simulink model "gm_sine_wave"  (R2020a)
settings: Solver=VariableStepAuto  StartTime=0.0  StopTime=1e-3  RelTol=1e-3
undefined symbols (not defined in the file or in its folder): amplitud, main_frequency, PLL_FREQUENCY
libraries: dspsrcs4 x1
settings Model: Creator=giova  LastModifiedBy=giova
settings OptimizationCC: BlockReduction=off  ConditionallyExecuteInputs=off
settings DebuggingCC: InheritedTsInSrcMsg=none

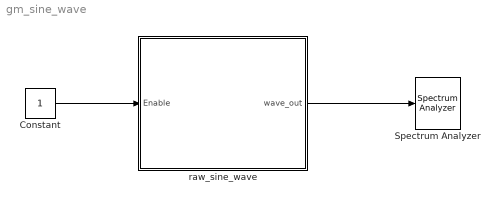
== system gm_sine_wave ==
  Constant : Constant  OutDataTypeStr=boolean  SampleTime=-1
  Spectrum Analyzer : SpectrumAnalyzer
  raw_sine_wave : Subsystem
  wires:
  Constant/1 -> raw_sine_wave/1(Enable)
  raw_sine_wave/1(wave_out) -> Spectrum Analyzer/1

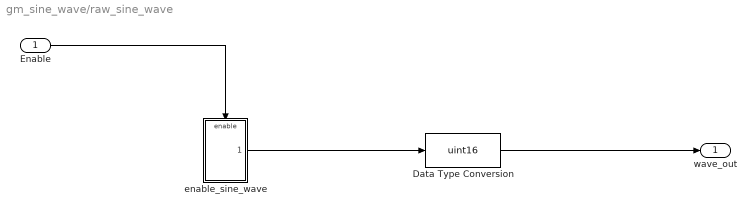
== system gm_sine_wave/raw_sine_wave ==
  Enable : Inport
  Data Type Conversion : DataTypeConversion  OutMin=0  OutMax=65535  OutDataTypeStr=uint16
  enable_sine_wave : Subsystem
  wave_out : Outport  InitialOutput=0
  wires:
  Data Type Conversion/1 -> wave_out/1
  enable_sine_wave/1(wave_out) -> Data Type Conversion/1
  Enable/1 -> enable_sine_wave/Enable

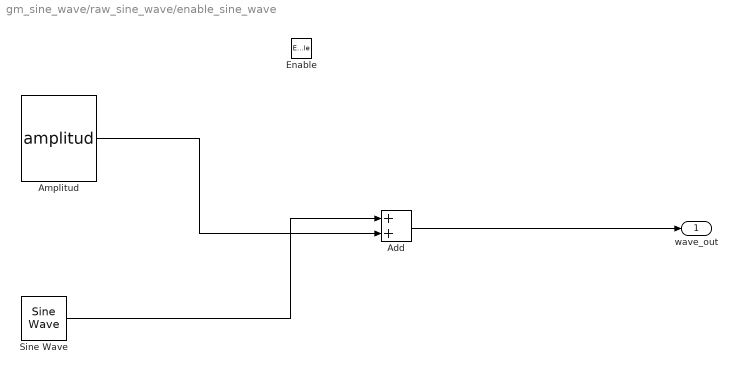
== system gm_sine_wave/raw_sine_wave/enable_sine_wave ==
  Enable : EnablePort
  Add : Sum
  Amplitud : Constant  Value=amplitud  OutDataTypeStr=fixdt(1,16)  SampleTime=-1
  Sine Wave : dspsrcs4/Sine Wave  Amplitude=amplitud  Frequency=main_frequency  Phase=0  SampleMode=Discrete  OutComplex=Real  CompMethod=Table lookup  TableSize=Speed  SampleTime=1/(PLL_FREQUENCY)  SamplesPerFrame=1  ResetState=Restart at time zero  OutputFrames=off  dataType=Fixed-point  wordLen=16  udDataType=sfix(16)  fracBitsMode=Best precision  numFracBits=14  OutDataTypeStr=fixdt(1,16)  LastOutDataTypeStr=fixdt(1,16)
  wave_out : Outport  InitialOutput=0
  wires:
  Add/1 -> wave_out/1
  Amplitud/1 -> Add/2
  Sine Wave/1 -> Add/1
